simulink model "gsm_blocks_eng"  (Simulink 6.0)
settings: Solver=VariableStepDiscrete  StartTime=0.0  StopTime=7  RelTol=1e-3
libraries: simulink x25, dspsigops x18, dspbuff3 x3, commchan2 x3, commcrc2 x2, commcnvcod2 x2, commblkintrlv2 x2, commsrccod2 x2, commdigbbndcpm2 x2, commrandsrc2 x1, commsink2 x1
settings Model: LastModifiedBy=Simón

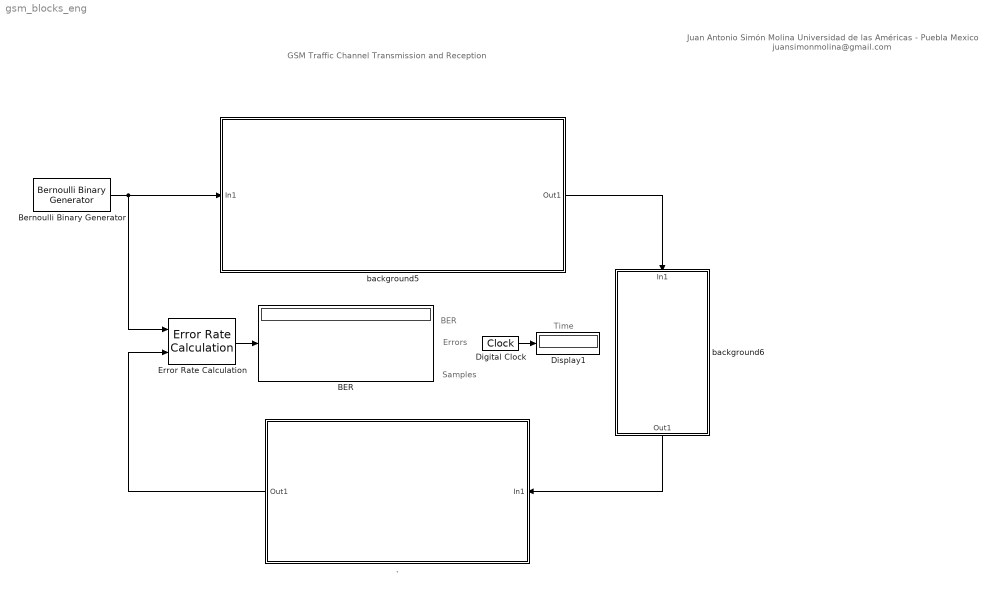
== system gsm_blocks_eng ==
  note: GSM Traffic Channel
      | Transmission and
      | Reception
  note: Juan Antonio Simón Molina
      | Universidad de las Américas - Puebla
      | Mexico
      | juansimonmolina@gmail.com
  note: Time
  note: BER
  note: Errors
  note: Samples
  . : Subsystem  Tag=Receiver  Orientation=left
      mask Display: disp('Receiver')
  BER : Display
  Bernoulli Binary Generator : commrandsrc2/Bernoulli Binary Generator  P=0.5  seed=11111  Ts=1/9600  frameBased=on  sampPerFrame=260  orient=off
  Digital Clock : DigitalClock  SampleTime=0.001
  Display1 : Display
  Error Rate Calculation : commsink2/Error Rate Calculation  N=0  st_delay=0  cp_mode=Entire frame  subframe=[]  PMode=Port  WsName=ErrorVec  RsMode2=off  stop=off  numErr=100  maxBits=1e6
  background5 : Subsystem  Tag=Transmitter
      mask Display: disp('Transmitter')
  background6 : Subsystem  Orientation=down
      mask Display: disp('Channel')
  wires:
  Bernoulli Binary Generator/1 -> background5/1(In1), Error Rate Calculation/1
  Error Rate Calculation/1 -> BER/1
  Digital Clock/1 -> Display1/1
  background5/1(Out1) -> background6/1(In1)
  ./1(Out1) -> Error Rate Calculation/2
  background6/1(Out1) -> ./1(In1)

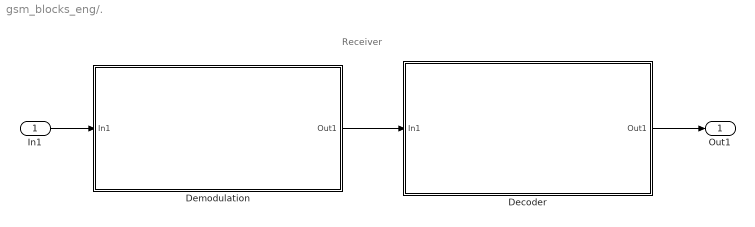
== system gsm_blocks_eng/. ==
  note: Receiver
  In1 : Inport  Port=1  LatchInput=off
  Decoder : Subsystem
      mask Display: disp('Decoder')
  Demodulation : Subsystem
      mask Display: disp('Demodulation')
  Out1 : Outport
  wires:
  In1/1 -> Demodulation/1(In1)
  Demodulation/1(Out1) -> Decoder/1(In1)
  Decoder/1(Out1) -> Out1/1

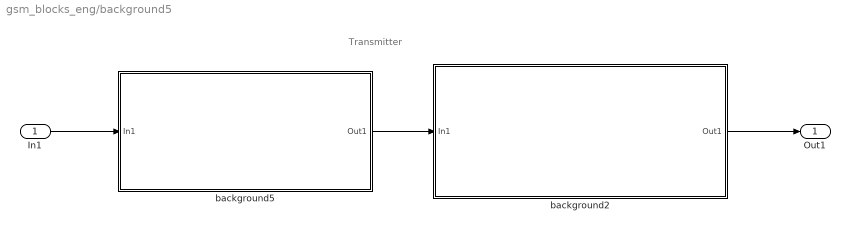
== system gsm_blocks_eng/background5 ==
  note: Transmitter
  In1 : Inport  Port=1  LatchInput=off
  background2 : Subsystem
      mask Display: disp('Modulation')
  background5 : Subsystem  Tag=Codificación
      mask Display: disp('Coding')
  Out1 : Outport
  wires:
  background5/1(Out1) -> background2/1(In1)
  background2/1(Out1) -> Out1/1
  In1/1 -> background5/1(In1)

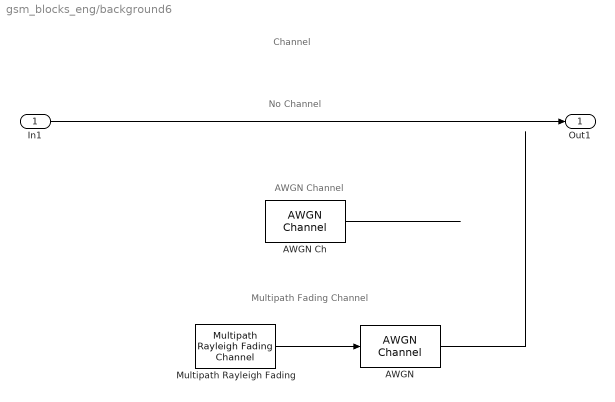
== system gsm_blocks_eng/background6 ==
  note: Channel
  note: No Channel
  note: AWGN Channel
  note: Multipath
      | Fading Channel
  In1 : Inport  Port=1  LatchInput=off
  AWGN : commchan2/AWGN Channel  seed=12345  noiseMode="Signal to noise ratio  (SNR)"  EbNodB=1  EsNodB=10  SNRdB=10  bitsPerSym=1  Ps=1e-3  Tsym=1/9600  variance=1
  AWGN Ch : commchan2/AWGN Channel  seed=67  noiseMode="Signal to noise ratio  (SNR)"  EbNodB=1  EsNodB=10  SNRdB=10  bitsPerSym=1  Ps=1e-3  Tsym=1/9600  variance=1
  Multipath Rayleigh Fading : commchan2/Multipath Rayleigh Fading Channel  Fd=50  simTs=260/(629*9600)  delayVec=[0 260e-9 521e-9 781e-9]  gainVecdB=[1 -3 -6 -9]  normGain=off  Seed=12345
  Out1 : Outport
  wires:
  Multipath Rayleigh Fading/1 -> AWGN/1
  ? -> AWGN Ch/1
  AWGN Ch/1 -> ?
  In1/1 -> Out1/1
  ? -> Multipath Rayleigh Fading/1
  AWGN/1 -> ?

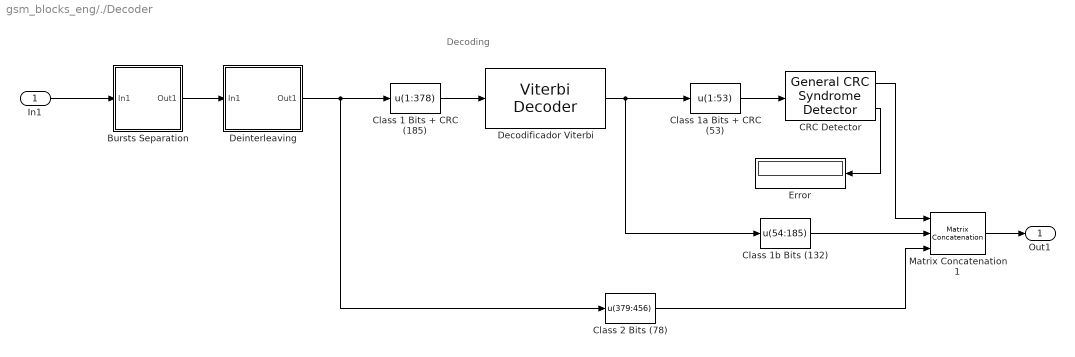
== system gsm_blocks_eng/./Decoder ==
  note: Decoding
  In1 : Inport  Port=1  LatchInput=off
  Bursts Separation : Subsystem
  CRC Detector : commcrc2/General CRC Syndrome Detector  genPoly=[1 1 0 1]  iniStates=[0]  numChecksums=1
  Class 1 Bits + CRC (185) : MATLABFcn  MATLABFcn=u(1:378)  OutputDimensions=[378,1]  Output1D=off
  Class 1a Bits + CRC (53) : MATLABFcn  MATLABFcn=u(1:53)  OutputDimensions=[53,1]  Output1D=off
  Class 1b Bits (132) : MATLABFcn  MATLABFcn=u(54:185)  OutputDimensions=[132,1]  Output1D=off
  Class 2 Bits (78) : MATLABFcn  MATLABFcn=u(379:456)  OutputDimensions=[78,1]  Output1D=off
  Decodificador Viterbi : commcnvcod2/Viterbi Decoder  trellis=poly2trellis(7, [133 171])  dectype=Hard Decision  nsdecb=4  tbdepth=10  opmode=Truncated  reset=off
  Deinterleaving : Subsystem
  Error : Display
  Matrix Concatenation1 : simulink/Math Operations/Matrix Concatenation  numInports=3  catMethod=Vertical
  Out1 : Outport
  wires:
  Deinterleaving/1(Out1) -> Class 1 Bits + CRC (185)/1, Class 2 Bits (78)/1
  Class 1 Bits + CRC (185)/1 -> Decodificador Viterbi/1
  Decodificador Viterbi/1 -> Class 1a Bits + CRC (53)/1, Class 1b Bits (132)/1
  Class 1a Bits + CRC (53)/1 -> CRC Detector/1
  Class 2 Bits (78)/1 -> Matrix Concatenation1/3
  Class 1b Bits (132)/1 -> Matrix Concatenation1/2
  CRC Detector/1 -> Matrix Concatenation1/1
  CRC Detector/2 -> Error/1
  Matrix Concatenation1/1 -> Out1/1
  Bursts Separation/1(Out1) -> Deinterleaving/1(In1)
  In1/1 -> Bursts Separation/1(In1)

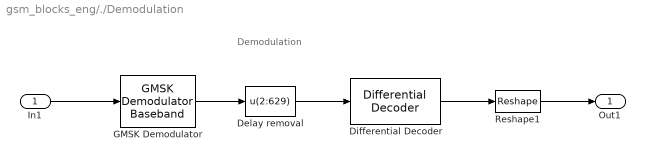
== system gsm_blocks_eng/./Demodulation ==
  note: Demodulation
  In1 : Inport  Port=1  LatchInput=off
  Delay removal : MATLABFcn  MATLABFcn=u(2:629)  OutputDimensions=[628,1]  Output1D=off
  Differential Decoder : commsrccod2/Differential Decoder  InitCond=0
  GMSK Demodulator : commdigbbndcpm2/GMSK Demodulator Baseband  OutputType=Bit  BT=.3  pulseLength=1  preHistory=1  phaseOffset=0  samplesPerSymbol=1  traceBack=1
  Reshape1 : simulink/Math Operations/Reshape  OutputDimensionality=Customize  OutputDimensions=[157,4]
  Out1 : Outport
  wires:
  In1/1 -> GMSK Demodulator/1
  GMSK Demodulator/1 -> Delay removal/1
  Differential Decoder/1 -> Reshape1/1
  Reshape1/1 -> Out1/1
  Delay removal/1 -> Differential Decoder/1

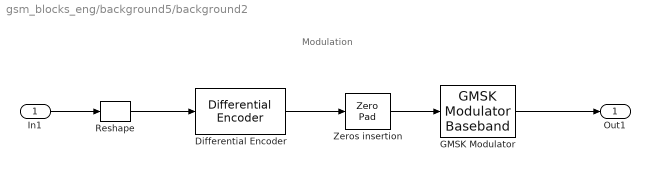
== system gsm_blocks_eng/background5/background2 ==
  note: Modulation
  In1 : Inport  Port=1  LatchInput=off
  Differential Encoder : commsrccod2/Differential Encoder  InitCond=0
  GMSK Modulator : commdigbbndcpm2/GMSK Modulator Baseband  inputType=Bit  BT=.3  pulseLength=1  preHistory=1  phaseOffset=0  samplesPerSymbol=1
  Reshape : simulink/Math Operations/Reshape  OutputDimensionality=Column vector  OutputDimensions=[1,1]
  Zeros insertion : dspsigops/Zero Pad  padSigAt=End  zpadAlong=Columns  padNumOutRowsSpecMethod=User-specified  numOutRows=629  padNumOutColsSpecMethod=User-specified  numOutCols=1  trunc_flag=None
  Out1 : Outport
  wires:
  Differential Encoder/1 -> Zeros insertion/1
  In1/1 -> Reshape/1
  GMSK Modulator/1 -> Out1/1
  Zeros insertion/1 -> GMSK Modulator/1
  Reshape/1 -> Differential Encoder/1

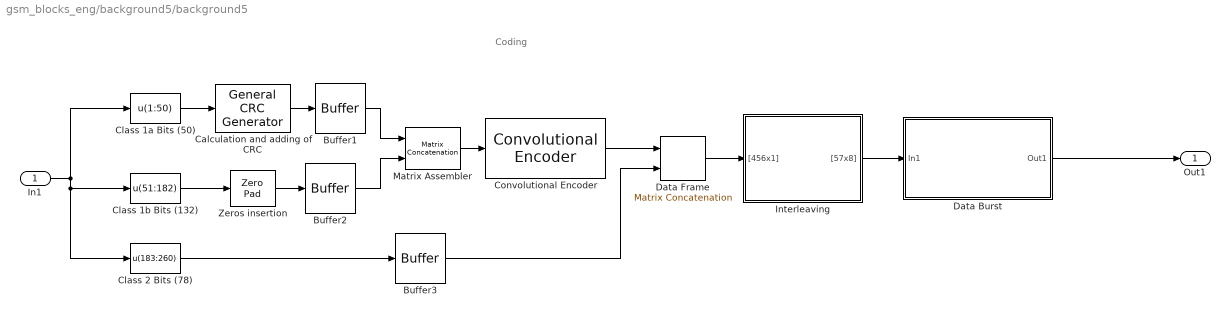
== system gsm_blocks_eng/background5/background5 ==
  note: Coding
  In1 : Inport  Port=1  LatchInput=off
  Buffer1 : dspbuff3/Buffer  N=53  V=0  ic=0
  Buffer2 : dspbuff3/Buffer  N=136  V=0  ic=0
  Buffer3 : dspbuff3/Buffer  N=78  V=0  ic=0
  Calculation and adding of CRC : commcrc2/General CRC Generator  genPoly=[1 1 0 1]  iniStates=[0]  numChecksums=1
  Class 1a Bits (50) : MATLABFcn  MATLABFcn=u(1:50)  OutputDimensions=[50,1]  Output1D=off
  Class 1b Bits (132) : MATLABFcn  MATLABFcn=u(51:182)  OutputDimensions=[132,1]  Output1D=off
  Class 2 Bits (78) : MATLABFcn  MATLABFcn=u(183:260)  OutputDimensions=[78,1]  Output1D=off
  Convolutional Encoder : commcnvcod2/Convolutional Encoder  trellis=poly2trellis(7,[133,171])  reset=None
  Data Burst : Subsystem
  "Data Frame " : simulink/Math Operations/Matrix Concatenation  numInports=2  catMethod=Vertical
  Interleaving : Subsystem
  Matrix Assembler : simulink/Math Operations/Matrix Concatenation  numInports=2  catMethod=Vertical
  Zeros insertion : dspsigops/Zero Pad  padSigAt=End  zpadAlong=Columns  padNumOutRowsSpecMethod=User-specified  numOutRows=136  padNumOutColsSpecMethod=User-specified  numOutCols=1  trunc_flag=None
  Out1 : Outport
  wires:
  Class 1a Bits (50)/1 -> Calculation and adding of CRC/1
  Calculation and adding of CRC/1 -> Buffer1/1
  Class 1b Bits (132)/1 -> Zeros insertion/1
  Class 2 Bits (78)/1 -> Buffer3/1
  Zeros insertion/1 -> Buffer2/1
  Matrix Assembler/1 -> Convolutional Encoder/1
  Convolutional Encoder/1 -> "Data Frame "/1
  Buffer1/1 -> Matrix Assembler/1
  Buffer2/1 -> Matrix Assembler/2
  Buffer3/1 -> "Data Frame "/2
  In1/1 -> Class 1a Bits (50)/1, Class 1b Bits (132)/1, Class 2 Bits (78)/1
  "Data Frame "/1 -> Interleaving/1("[456x1]")
  Interleaving/1("[57x8]") -> Data Burst/1(In1)
  Data Burst/1(Out1) -> Out1/1

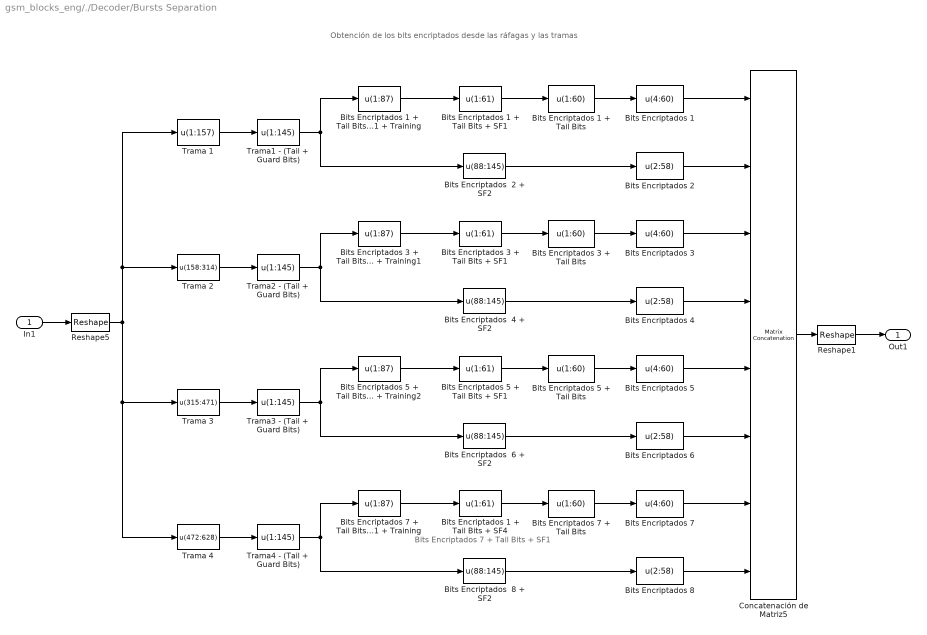
== system gsm_blocks_eng/./Decoder/Bursts Separation ==
  note: Obtención de los bits encriptados
      | desde las ráfagas y las tramas
  note: Bits Encriptados 7
      | + Tail Bits + SF1
  In1 : Inport  Port=1  LatchInput=off
  Bits Encriptados  2 + SF2 : MATLABFcn  MATLABFcn=u(88:145)  OutputDimensions=[58,1]  Output1D=off
  Bits Encriptados  4 + SF2 : MATLABFcn  MATLABFcn=u(88:145)  OutputDimensions=[58,1]  Output1D=off
  Bits Encriptados  6 + SF2 : MATLABFcn  MATLABFcn=u(88:145)  OutputDimensions=[58,1]  Output1D=off
  Bits Encriptados  8 + SF2 : MATLABFcn  MATLABFcn=u(88:145)  OutputDimensions=[58,1]  Output1D=off
  Bits Encriptados {1,3,5,7} (4 alike) : MATLABFcn  MATLABFcn=u(4:60)  OutputDimensions=[57,1]  Output1D=off
  Bits Encriptados 1 + Tail Bits : MATLABFcn  MATLABFcn=u(1:60)  OutputDimensions=[60,1]  Output1D=off
  Bits Encriptados 1 + Tail Bits + SF1 : MATLABFcn  MATLABFcn=u(1:61)  OutputDimensions=[61,1]  Output1D=off
  Bits Encriptados 1 + Tail Bits + SF4 : MATLABFcn  MATLABFcn=u(1:61)  OutputDimensions=[61,1]  Output1D=off
  Bits Encriptados 1 + Tail Bits + SF1 + Training : MATLABFcn  MATLABFcn=u(1:87)  OutputDimensions=[87,1]  Output1D=off
  Bits Encriptados {2,4,6,8} (4 alike) : MATLABFcn  MATLABFcn=u(2:58)  OutputDimensions=[57,1]  Output1D=off
  Bits Encriptados 3 + Tail Bits : MATLABFcn  MATLABFcn=u(1:60)  OutputDimensions=[60,1]  Output1D=off
  Bits Encriptados 3 + Tail Bits + SF1 : MATLABFcn  MATLABFcn=u(1:61)  OutputDimensions=[61,1]  Output1D=off
  Bits Encriptados 3 + Tail Bits + SF1 + Training1 : MATLABFcn  MATLABFcn=u(1:87)  OutputDimensions=[87,1]  Output1D=off
  Bits Encriptados 5 + Tail Bits : MATLABFcn  MATLABFcn=u(1:60)  OutputDimensions=[60,1]  Output1D=off
  Bits Encriptados 5 + Tail Bits + SF1 : MATLABFcn  MATLABFcn=u(1:61)  OutputDimensions=[61,1]  Output1D=off
  Bits Encriptados 5 + Tail Bits + SF1 + Training2 : MATLABFcn  MATLABFcn=u(1:87)  OutputDimensions=[87,1]  Output1D=off
  Bits Encriptados 7 + Tail Bits : MATLABFcn  MATLABFcn=u(1:60)  OutputDimensions=[60,1]  Output1D=off
  Bits Encriptados 7 + Tail Bits + SF1 + Training : MATLABFcn  MATLABFcn=u(1:87)  OutputDimensions=[87,1]  Output1D=off
  Concatenación de Matriz5 : simulink/Math Operations/Matrix Concatenation  numInports=8  catMethod=Vertical
  Reshape1 : simulink/Math Operations/Reshape  OutputDimensionality=Customize  OutputDimensions=[57,8]
  Reshape5 : simulink/Math Operations/Reshape  OutputDimensionality=Column vector  OutputDimensions=[157,4]
  Trama 1 : MATLABFcn  MATLABFcn=u(1:157)  OutputDimensions=[157,1]  Output1D=off
  Trama 2 : MATLABFcn  MATLABFcn=u(158:314)  OutputDimensions=[157,1]  Output1D=off
  Trama 3 : MATLABFcn  MATLABFcn=u(315:471)  OutputDimensions=[157,1]  Output1D=off
  Trama 4 : MATLABFcn  MATLABFcn=u(472:628)  OutputDimensions=[157,1]  Output1D=off
  Trama1 - (Tail + Guard Bits) : MATLABFcn  MATLABFcn=u(1:145)  OutputDimensions=[145,1]  Output1D=off
  Trama2 - (Tail + Guard Bits) : MATLABFcn  MATLABFcn=u(1:145)  OutputDimensions=[145,1]  Output1D=off
  Trama3 - (Tail + Guard Bits) : MATLABFcn  MATLABFcn=u(1:145)  OutputDimensions=[145,1]  Output1D=off
  Trama4 - (Tail + Guard Bits) : MATLABFcn  MATLABFcn=u(1:145)  OutputDimensions=[145,1]  Output1D=off
  Out1 : Outport
  wires:
  In1/1 -> Reshape5/1
  Reshape5/1 -> Trama 1/1, Trama 2/1, Trama 4/1, Trama 3/1
  Trama 1/1 -> Trama1 - (Tail + Guard Bits)/1
  Trama1 - (Tail + Guard Bits)/1 -> Bits Encriptados  2 + SF2/1, Bits Encriptados 1 + Tail Bits + SF1 + Training/1
  Bits Encriptados 1 + Tail Bits + SF1 + Training/1 -> Bits Encriptados 1 + Tail Bits + SF1/1
  Bits Encriptados 1 + Tail Bits + SF1/1 -> Bits Encriptados 1 + Tail Bits/1
  Bits Encriptados 1 + Tail Bits/1 -> Bits Encriptados 1/1
  Bits Encriptados  2 + SF2/1 -> Bits Encriptados 2/1
  Trama 2/1 -> Trama2 - (Tail + Guard Bits)/1
  Trama2 - (Tail + Guard Bits)/1 -> Bits Encriptados  4 + SF2/1, Bits Encriptados 3 + Tail Bits + SF1 + Training1/1
  Bits Encriptados 3 + Tail Bits + SF1 + Training1/1 -> Bits Encriptados 3 + Tail Bits + SF1/1
  Bits Encriptados 3 + Tail Bits + SF1/1 -> Bits Encriptados 3 + Tail Bits/1
  Bits Encriptados 3 + Tail Bits/1 -> Bits Encriptados 3/1
  Bits Encriptados  4 + SF2/1 -> Bits Encriptados 4/1
  Trama 3/1 -> Trama3 - (Tail + Guard Bits)/1
  Trama3 - (Tail + Guard Bits)/1 -> Bits Encriptados  6 + SF2/1, Bits Encriptados 5 + Tail Bits + SF1 + Training2/1
  Bits Encriptados 5 + Tail Bits + SF1 + Training2/1 -> Bits Encriptados 5 + Tail Bits + SF1/1
  Bits Encriptados 5 + Tail Bits + SF1/1 -> Bits Encriptados 5 + Tail Bits/1
  Bits Encriptados 5 + Tail Bits/1 -> Bits Encriptados 5/1
  Bits Encriptados  6 + SF2/1 -> Bits Encriptados 6/1
  Trama 4/1 -> Trama4 - (Tail + Guard Bits)/1
  Trama4 - (Tail + Guard Bits)/1 -> Bits Encriptados  8 + SF2/1, Bits Encriptados 7 + Tail Bits + SF1 + Training/1
  Bits Encriptados 7 + Tail Bits + SF1 + Training/1 -> Bits Encriptados 1 + Tail Bits + SF4/1
  Bits Encriptados 1 + Tail Bits + SF4/1 -> Bits Encriptados 7 + Tail Bits/1
  Bits Encriptados 7 + Tail Bits/1 -> Bits Encriptados 7/1
  Bits Encriptados  8 + SF2/1 -> Bits Encriptados 8/1
  Bits Encriptados 1/1 -> Concatenación de Matriz5/1
  Bits Encriptados 2/1 -> Concatenación de Matriz5/2
  Bits Encriptados 3/1 -> Concatenación de Matriz5/3
  Bits Encriptados 4/1 -> Concatenación de Matriz5/4
  Bits Encriptados 5/1 -> Concatenación de Matriz5/5
  Bits Encriptados 6/1 -> Concatenación de Matriz5/6
  Bits Encriptados 7/1 -> Concatenación de Matriz5/7
  Bits Encriptados 8/1 -> Concatenación de Matriz5/8
  Concatenación de Matriz5/1 -> Reshape1/1
  Reshape1/1 -> Out1/1

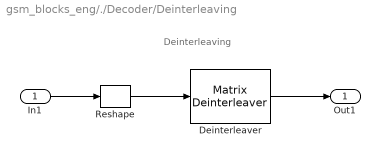
== system gsm_blocks_eng/./Decoder/Deinterleaving ==
  note: Deinterleaving
  In1 : Inport  Port=1  LatchInput=off
  Deinterleaver : commblkintrlv2/Matrix Deinterleaver  Nrows=57  Ncols=8
  Reshape : simulink/Math Operations/Reshape  OutputDimensionality=Column vector  OutputDimensions=[1,1]
  Out1 : Outport
  wires:
  In1/1 -> Reshape/1
  Deinterleaver/1 -> Out1/1
  Reshape/1 -> Deinterleaver/1

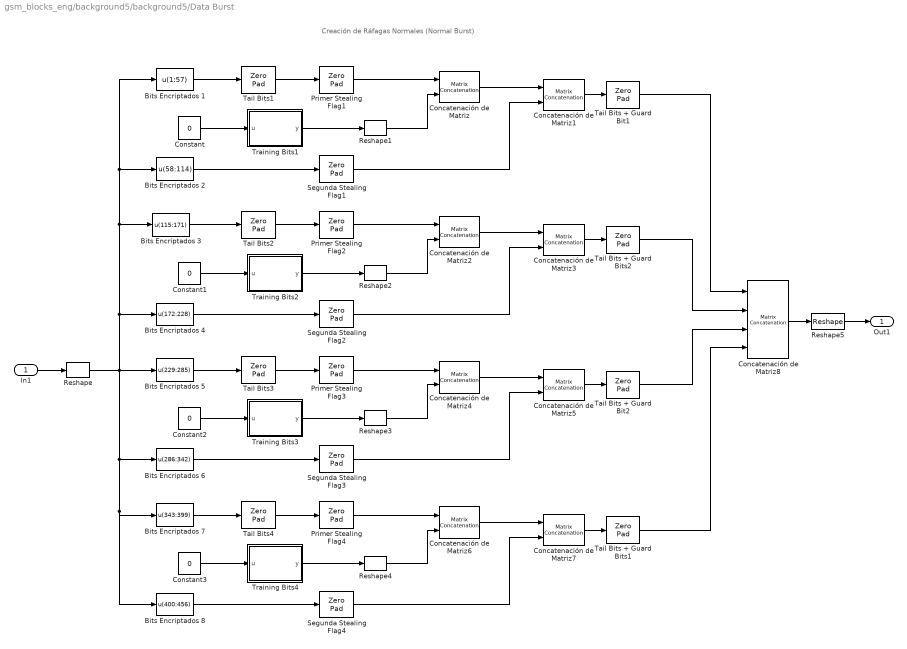
== system gsm_blocks_eng/background5/background5/Data Burst ==
  note: Creación de Ráfagas Normales
      | (Normal Burst)
  In1 : Inport  Port=1  LatchInput=off
  Bits Encriptados 1 : MATLABFcn  MATLABFcn=u(1:57)  OutputDimensions=[57,1]  Output1D=off
  Bits Encriptados 2 : MATLABFcn  MATLABFcn=u(58:114)  OutputDimensions=[57,1]  Output1D=off
  Bits Encriptados 3 : MATLABFcn  MATLABFcn=u(115:171)  OutputDimensions=[57,1]  Output1D=off
  Bits Encriptados 4 : MATLABFcn  MATLABFcn=u(172:228)  OutputDimensions=[57,1]  Output1D=off
  Bits Encriptados 5 : MATLABFcn  MATLABFcn=u(229:285)  OutputDimensions=[57,1]  Output1D=off
  Bits Encriptados 6 : MATLABFcn  MATLABFcn=u(286:342)  OutputDimensions=[57,1]  Output1D=off
  Bits Encriptados 7 : MATLABFcn  MATLABFcn=u(343:399)  OutputDimensions=[57,1]  Output1D=off
  Bits Encriptados 8 : MATLABFcn  MATLABFcn=u(400:456)  OutputDimensions=[57,1]  Output1D=off
  Concatenación de Matriz{,1..7} (8 alike) : simulink/Math Operations/Matrix Concatenation  numInports=2  catMethod=Vertical
  Concatenación de Matriz8 : simulink/Math Operations/Matrix Concatenation  numInports=4  catMethod=Vertical
  Constant{,1..3} (4 alike) : Constant  Value=0
  Primer Stealing Flag{1..4} (4 alike) : dspsigops/Zero Pad  padSigAt=End  zpadAlong=Columns  padNumOutRowsSpecMethod=User-specified  numOutRows=61  padNumOutColsSpecMethod=User-specified  numOutCols=1  trunc_flag=None
  Reshape{,1..4} (5 alike) : simulink/Math Operations/Reshape  OutputDimensionality=Column vector  OutputDimensions=[1,1]
  Reshape5 : simulink/Math Operations/Reshape  OutputDimensionality=Customize  OutputDimensions=[157,4]
  Segunda Stealing Flag{1..4} (4 alike) : dspsigops/Zero Pad  padSigAt=Beginning  zpadAlong=Columns  padNumOutRowsSpecMethod=User-specified  numOutRows=58  padNumOutColsSpecMethod=User-specified  numOutCols=1  trunc_flag=None
  Tail Bits + Guard Bit1 : dspsigops/Zero Pad  padSigAt=End  zpadAlong=Columns  padNumOutRowsSpecMethod=User-specified  numOutRows=157  padNumOutColsSpecMethod=User-specified  numOutCols=1  trunc_flag=None
  Tail Bits + Guard Bit2 : dspsigops/Zero Pad  padSigAt=End  zpadAlong=Columns  padNumOutRowsSpecMethod=User-specified  numOutRows=157  padNumOutColsSpecMethod=User-specified  numOutCols=1  trunc_flag=None
  Tail Bits + Guard Bits1 : dspsigops/Zero Pad  padSigAt=End  zpadAlong=Columns  padNumOutRowsSpecMethod=User-specified  numOutRows=157  padNumOutColsSpecMethod=User-specified  numOutCols=1  trunc_flag=None
  Tail Bits + Guard Bits2 : dspsigops/Zero Pad  padSigAt=End  zpadAlong=Columns  padNumOutRowsSpecMethod=User-specified  numOutRows=157  padNumOutColsSpecMethod=User-specified  numOutCols=1  trunc_flag=None
  Tail Bits{1..4} (4 alike) : dspsigops/Zero Pad  padSigAt=Beginning  zpadAlong=Columns  padNumOutRowsSpecMethod=User-specified  numOutRows=60  padNumOutColsSpecMethod=User-specified  numOutCols=1  trunc_flag=None
  Training Bits1 : Stateflow chart
  Training Bits2 : Stateflow chart
  Training Bits3 : Stateflow chart
  Training Bits4 : Stateflow chart
  Out1 : Outport
  wires:
  In1/1 -> Reshape/1
  Reshape/1 -> Bits Encriptados 1/1, Bits Encriptados 2/1, Bits Encriptados 3/1, Bits Encriptados 4/1, Bits Encriptados 5/1, Bits Encriptados 8/1, Bits Encriptados 7/1, Bits Encriptados 6/1
  Bits Encriptados 1/1 -> Tail Bits1/1
  Tail Bits1/1 -> Primer Stealing Flag1/1
  Training Bits1/1(y) -> Reshape1/1
  Reshape1/1 -> Concatenación de Matriz/2
  Constant/1 -> Training Bits1/1(u)
  Bits Encriptados 2/1 -> Segunda Stealing Flag1/1
  Concatenación de Matriz/1 -> Concatenación de Matriz1/1
  Concatenación de Matriz1/1 -> Tail Bits + Guard Bit1/1
  Primer Stealing Flag1/1 -> Concatenación de Matriz/1
  Segunda Stealing Flag1/1 -> Concatenación de Matriz1/2
  Bits Encriptados 3/1 -> Tail Bits2/1
  Tail Bits2/1 -> Primer Stealing Flag2/1
  Training Bits2/1(y) -> Reshape2/1
  Reshape2/1 -> Concatenación de Matriz2/2
  Constant1/1 -> Training Bits2/1(u)
  Bits Encriptados 4/1 -> Segunda Stealing Flag2/1
  Concatenación de Matriz2/1 -> Concatenación de Matriz3/1
  Concatenación de Matriz3/1 -> Tail Bits + Guard Bits2/1
  Primer Stealing Flag2/1 -> Concatenación de Matriz2/1
  Segunda Stealing Flag2/1 -> Concatenación de Matriz3/2
  Bits Encriptados 5/1 -> Tail Bits3/1
  Tail Bits3/1 -> Primer Stealing Flag3/1
  Training Bits3/1(y) -> Reshape3/1
  Reshape3/1 -> Concatenación de Matriz4/2
  Constant2/1 -> Training Bits3/1(u)
  Bits Encriptados 6/1 -> Segunda Stealing Flag3/1
  Concatenación de Matriz4/1 -> Concatenación de Matriz5/1
  Concatenación de Matriz5/1 -> Tail Bits + Guard Bit2/1
  Primer Stealing Flag3/1 -> Concatenación de Matriz4/1
  Segunda Stealing Flag3/1 -> Concatenación de Matriz5/2
  Bits Encriptados 7/1 -> Tail Bits4/1
  Tail Bits4/1 -> Primer Stealing Flag4/1
  Training Bits4/1(y) -> Reshape4/1
  Reshape4/1 -> Concatenación de Matriz6/2
  Constant3/1 -> Training Bits4/1(u)
  Bits Encriptados 8/1 -> Segunda Stealing Flag4/1
  Concatenación de Matriz6/1 -> Concatenación de Matriz7/1
  Concatenación de Matriz7/1 -> Tail Bits + Guard Bits1/1
  Primer Stealing Flag4/1 -> Concatenación de Matriz6/1
  Segunda Stealing Flag4/1 -> Concatenación de Matriz7/2
  Tail Bits + Guard Bit1/1 -> Concatenación de Matriz8/1
  Tail Bits + Guard Bits2/1 -> Concatenación de Matriz8/2
  Tail Bits + Guard Bit2/1 -> Concatenación de Matriz8/3
  Tail Bits + Guard Bits1/1 -> Concatenación de Matriz8/4
  Concatenación de Matriz8/1 -> Reshape5/1
  Reshape5/1 -> Out1/1

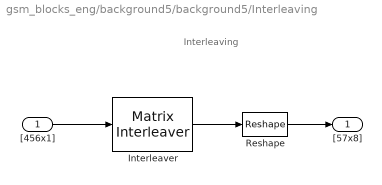
== system gsm_blocks_eng/background5/background5/Interleaving ==
  note: Interleaving
  "[456x1]" : Inport  Port=1  LatchInput=off
  Interleaver : commblkintrlv2/Matrix Interleaver  Nrows=57  Ncols=8
  Reshape : simulink/Math Operations/Reshape  OutputDimensionality=Customize  OutputDimensions=[57,8]
  "[57x8]" : Outport
  wires:
  "[456x1]"/1 -> Interleaver/1
  Interleaver/1 -> Reshape/1
  Reshape/1 -> "[57x8]"/1

== matlab function background5/background5/Data Burst/Training Bits2 ==
  data: u input inherited; y output inherited
function y = fcn(u)
% This block supports an embeddable subset of the MATLAB language.
% See the help menu for details. 

training2 = [0,0,1,0,1,1,0,1,1,1,0,1,1,1,1,0,0,0,1,0,1,1,0,1,1,1];
y = training2;

== matlab function background5/background5/Data Burst/Training Bits1 ==
  data: u input inherited; y output inherited
function y = fcn(u)
% This block supports an embeddable subset of the MATLAB language.
% See the help menu for details. 

training1 = [0,0,1,0,0,1,0,1,1,1,0,0,0,0,1,0,0,0,1,0,0,1,0,1,1,1];
y = training1;

== matlab function background5/background5/Data Burst/Training Bits3 ==
  data: u input inherited; y output inherited
function y = fcn(u)
% This block supports an embeddable subset of the MATLAB language.
% See the help menu for details. 

training3 = [0,1,0,0,0,0,1,1,1,0,1,1,1,0,1,0,0,1,0,0,0,0,1,1,1,0];
y = training3;

== matlab function background5/background5/Data Burst/Training Bits4 ==
  data: u input inherited; y output inherited
function y = fcn(u)
% This block supports an embeddable subset of the MATLAB language.
% See the help menu for details. 

training4 = [0,1,0,0,0,1,1,1,1,0,1,1,0,1,0,0,0,1,0,0,0,1,1,1,1,0];
y = training4;
